simulink model "LQG_tw_v3"  (R2019a)
settings: Solver=FixedStepAuto  StartTime=0.0  StopTime=15  FixedStep=0.01  RelTol=1e-3
undefined symbols (not defined in the file): A, B, C, K, L
libraries: simulink x3, simulink_extras x1
settings Model: Creator=chute  LastModifiedBy=chute
settings DataIOCC: ReturnWorkspaceOutputs=off

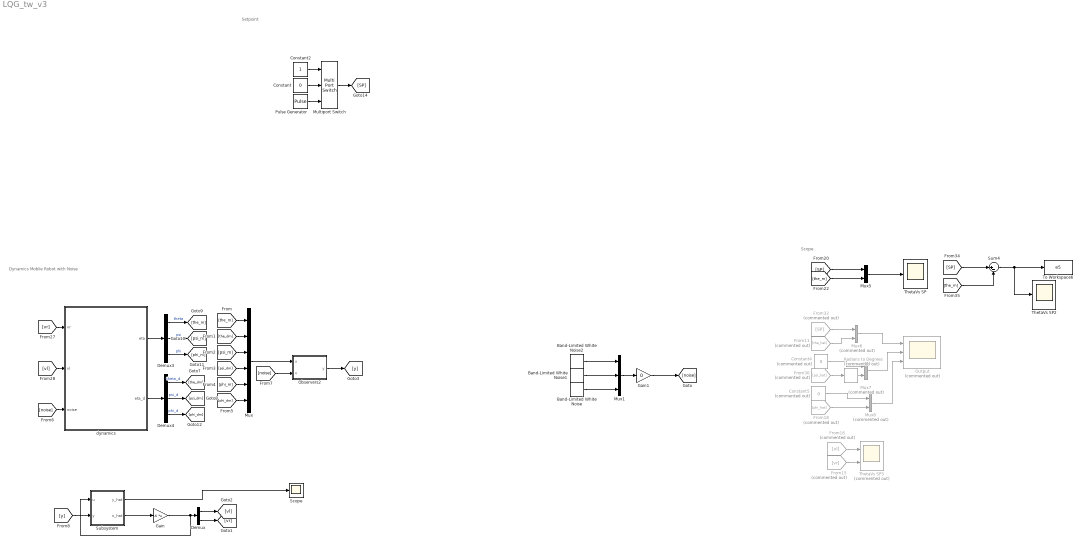
== system LQG_tw_v3 ==
  note: Scope
  note: Setpoint
  note: Dynamics Moblie Robot with Noise
  Band-Limited White Noise : simulink/Sources/Band-Limited White Noise  Cov=[0.0001]  Ts=0.1  seed=[23341]
  Band-Limited White Noise1 : simulink/Sources/Band-Limited White Noise  Cov=[0.0001]  Ts=0.1  seed=[23341]
  Band-Limited White Noise2 : simulink/Sources/Band-Limited White Noise  Cov=[0.1]  Ts=0.1  seed=[23341]
  Constant : Constant  Value=0
  Constant2 : Constant
  Constant4 : Constant  Commented=on  Value=0
  Constant5 : Constant  Commented=on  Value=0
  Demux : Demux  Outputs=2
  Demux3 : Demux  Outputs=3
  Demux4 : Demux  Outputs=3
  From11 : From  Commented=on  GotoTag=the_hat
  From15 : From  Commented=on  GotoTag=vr
  From16 : From  Commented=on  GotoTag=vl
  From18 : From  Commented=on  GotoTag=phi_hat
  From30 : From  Commented=on  GotoTag=psi_hat
  From32 : From  Commented=on  GotoTag=SP
  Gain : Gain  Gain=-K  Multiplication=Matrix(K*u)
  Gain1 : Gain  Gain=0
  Multiport Switch : MultiPortSwitch  Inputs=2
  Mux : Mux  Inputs=6
  Mux1 : Mux  Inputs=3
  Mux5 : Mux  Inputs=2
  Mux6 : Mux  Commented=on  Inputs=2
  Mux7 : Mux  Commented=on  Inputs=2
  Mux8 : Mux  Commented=on  Inputs=2
  Observers2 : MATLAB Function  TreatAsAtomicUnit=on
  Output : Scope  Commented=on  NumInputPorts=3
  Pulse Generator : DiscretePulseGenerator  PulseType=Time based  Amplitude=3.14  Period=10  PulseWidth=50
  Radians to Degrees : simulink_extras/Transformations/Radians to Degrees  Commented=on
  Scope : Scope
  Subsystem : Subsystem
  Sum4 : Sum  Inputs=|+-
  ThetaVs SP : Scope
  ThetaVs SP2 : Scope
  ThetaVs SP3 : Scope  Commented=on  NumInputPorts=2
  To Workspace6 : ToWorkspace  VariableName=e5  SaveFormat=Structure With Time  SampleTime=-1
  dynamics : Subsystem
  wires:
  dynamics/1(eta) -> Demux3/1
  Demux4/1 -> [the_dm]  "theta_d"
  dynamics/2(eta_d) -> Demux4/1
  Demux4/3 -> [phi_dm]  "phi_d"
  Demux4/2 -> [psi_dm]  "psi_d"
  Multiport Switch/1 -> [SP]
  Constant/1 -> Multiport Switch/2
  Constant2/1 -> Multiport Switch/1
  Mux5/1 -> ThetaVs SP/1
  [SP] -> Mux5/1
  [the_m] -> Mux5/2
  Demux3/3 -> [phi_m]  "phi"
  Demux3/2 -> [psi_m]  "psi"
  Demux3/1 -> [the_m]  "theta"
  [vl] -> dynamics/2("vl ")
  [vr] -> dynamics/1(vr)
  Mux8/1 -> Output/3
  Mux7/1 -> Output/2
  Mux6/1 -> Output/1
  From11/1 -> Mux6/2
  From32/1 -> Mux6/1
  From30/1 -> Radians to Degrees/1
  Constant4/1 -> Mux7/1
  Constant5/1 -> Mux8/1
  [SP] -> Sum4/1
  [the_m] -> Sum4/2
  Sum4/1 -> ThetaVs SP2/1, To Workspace6/1
  Pulse Generator/1 -> Multiport Switch/3
  [noise] -> dynamics/3(noise)
  Radians to Degrees/1 -> Mux7/2
  From16/1 -> ThetaVs SP3/1
  From15/1 -> ThetaVs SP3/2
  From18/1 -> Mux8/2
  Observers2/1(y) -> [y]
  [the_dm] -> Mux/2
  [the_m] -> Mux/1
  [psi_m] -> Mux/3
  [psi_dm] -> Mux/4
  [phi_m] -> Mux/5
  [phi_dm] -> Mux/6
  Mux/1 -> Observers2/1(x)
  Band-Limited White Noise2/1 -> Mux1/1
  Band-Limited White Noise1/1 -> Mux1/2
  Band-Limited White Noise/1 -> Mux1/3
  Mux1/1 -> Gain1/1
  [noise] -> Observers2/2(v)
  Subsystem/2(x_hat) -> Gain/1
  Gain/1 -> Subsystem/1("u "), Demux/1
  Demux/2 -> [vr]
  Demux/1 -> [vl]
  Subsystem/1(y_hat) -> Scope/1
  Gain1/1 -> [noise]
  [y] -> Subsystem/2(y)

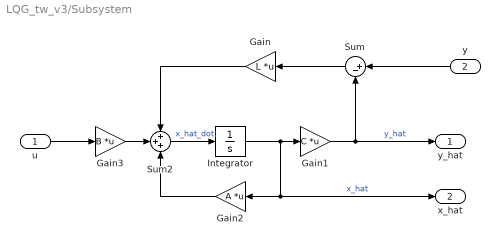
== system LQG_tw_v3/Subsystem ==
  "u " : Inport
  y : Inport  Port=2
  Gain : Gain  Gain=L  Multiplication=Matrix(K*u) (u vector)
  Gain1 : Gain  Gain=C  Multiplication=Matrix(K*u)
  Gain2 : Gain  Gain=A  Multiplication=Matrix(K*u)
  Gain3 : Gain  Gain=B  Multiplication=Matrix(K*u)
  Integrator : Integrator
  Sum : Sum  Inputs=|+-
  Sum2 : Sum  Inputs=+++
  y_hat : Outport
  x_hat : Outport  Port=2
  wires:
  Gain3/1 -> Sum2/2
  Gain2/1 -> Sum2/3
  Integrator/1 -> x_hat/1, Gain2/1, Gain1/1  "x_hat"
  Gain1/1 -> y_hat/1, Sum/2  "y_hat"
  Sum2/1 -> Integrator/1  "x_hat_dot"
  y/1 -> Sum/1
  Gain/1 -> Sum2/1
  Sum/1 -> Gain/1
  "u "/1 -> Gain3/1

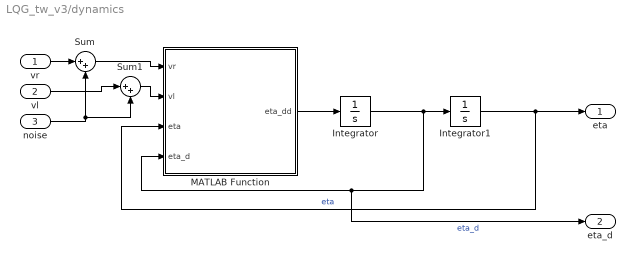
== system LQG_tw_v3/dynamics ==
  vr : Inport
  "vl " : Inport  Port=2
  noise : Inport  Port=3
  Integrator : Integrator  InitialCondition=[0;0;0]
  Integrator1 : Integrator  InitialCondition=[0;0.3*pi/180;0]
  MATLAB Function : MATLAB Function  TreatAsAtomicUnit=on
  Sum : Sum  Inputs=|++
  Sum1 : Sum  Inputs=|++
  eta : Outport
  eta_d : Outport  Port=2
  wires:
  Integrator/1 -> Integrator1/1, eta_d/1, MATLAB Function/4(eta_d)  "eta_d"
  Integrator1/1 -> eta/1, MATLAB Function/3(eta)  "eta"
  MATLAB Function/1(eta_dd) -> Integrator/1
  vr/1 -> Sum/1
  Sum/1 -> MATLAB Function/1(vr)
  Sum1/1 -> MATLAB Function/2(vl)
  "vl "/1 -> Sum1/1
  noise/1 -> Sum1/2, Sum/2

== matlab function LQG_tw_v3/Observers2 ==
  data: x input; y output; v input
function y= fcn(x,v)
C = [1 0 0 0 0 0; 
     0 0 1 0 0 0;
     0 0 0 0 1 0];

y = C*x+v;
end

== matlab function LQG_tw_v3/dynamics/MATLAB Function ==
  data: vr input; vl input; eta_dd output; eta input; eta_d input
function eta_dd= fcn(vr,vl,eta,eta_d)
%% declare the parameter:
%% Hoang

g =9.81; % gravity acceleration
m =0.046; % wheel weight
R =0.0335; % Wheel radius
M =0.945;  % body weight
W =0.17; % Body width
D =0.1; % Body depth
H =0.121;% Body Height
L =0.121/2;% distance

n =30 ; %gear ratio
Rm=8.0013;      %dien tro dong co DC
Kb=0.45096;   %he so emf cua dong co
Kt=0.45096;   %momemt xoan cua dong co DC\
fm = 0.21895; % friction cof between body and DC motor.
fw = 0.01; % friction cof between wheel and floor
anp = (n*Kt)/Rm;
bet = (n*Kt*Kb/Rm)+fm;

J_psi  = M*L^2/3; % Body inertia moment
Jw = m*R^2/2;  %Wheel inertia moment
J_phi = M*(W^2+D^2)/12; % Body yaw inertia moment
Jm = 0.00083134;
anp = (n*Kt)/Rm;
bet = (n*Kt*Kb/Rm)+fm;

%% Notation:
the=eta(1,1);
psi=eta(2,1);
phi=eta(3,1);

the_dot=eta_d(1,1);
psi_dot=eta_d(2,1);
phi_dot=eta_d(3,1);

tor=[vl;vr];



%% DC Motor
F_the = anp*(vl+vr)-2*(bet+fw)*the_dot+2*bet*psi_dot;
F_psi = -anp*(vl+vr)+2*bet*the_dot-2*bet*psi_dot;
F_phi = W*anp*(vr-vl)/(2*R)-W^2*((bet+fw)*phi_dot)/2*R^2;
tor =[F_the;F_psi;F_phi];

%% dyn
% Mass matrix:
M1 = ...
[2*Jw + 2*Jm*n^2 + R^2*(M + 2*m),L*M*R*cos(psi) - 2*Jm*n^2,0;
 L*M*R*cos(psi) - 2*Jm*n^2,J_psi + L^2*M + 2*Jm*n^2,0;
 0,0,J_phi + (W^2*m)/2 + L^2*M*sin(psi)^2 + (W^2*(Jw + Jm*n^2))/(2*R^2)];

%Coriolis matrix:
C1 = ...
[0,-L*M*R*psi_dot*sin(psi),0;
 0,0,-(L^2*M*phi_dot*sin(2*psi))/2;
 0,(L^2*M*phi_dot*sin(2*psi))/2,(L^2*M*psi_dot*sin(2*psi))/2];


% Gravity vector:
G1=...
[0;
-L*M*g*sin(psi);
0];
%% Input Matrices:
% B1=[1/R,        1/R;
%     -1,          -1;
%     W/(2*R),-W/(2*R)];

%% External Force

eta_dd=inv(M1)*(tor-C1*eta_d-G1);
end
